simulink model "sampleModel54"  (R2021a)
settings: Solver=VariableStepAuto  StartTime=0.0  StopTime=10.0  RelTol=1e-3
libraries: simulink x28, simulink_need_slupdate x2
settings Model: Creator=user  LastModifiedBy=user

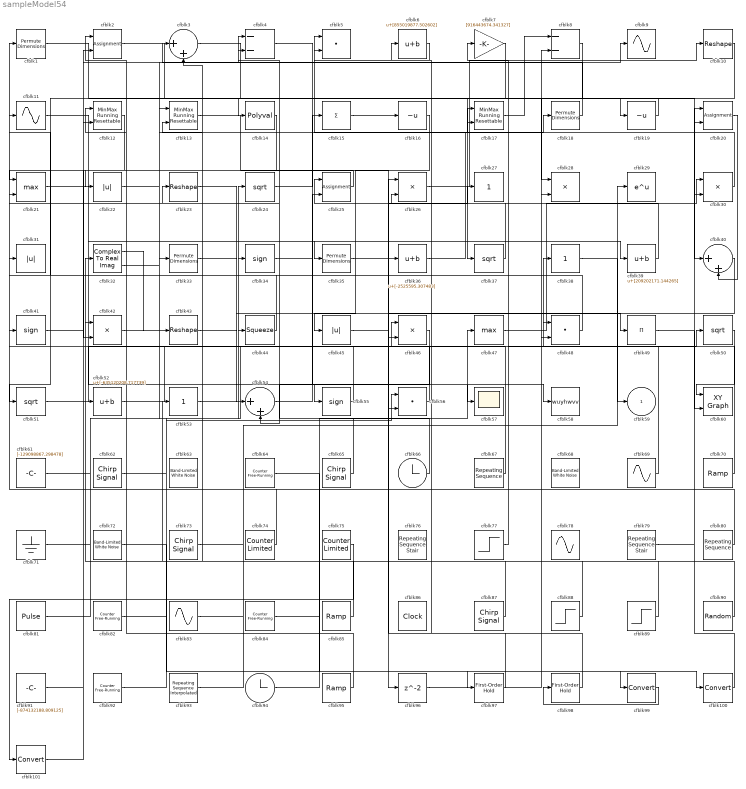
== system sampleModel54 ==
  cfblk{1,18,33,35} (4 alike) : PermuteDimensions
  cfblk10 : Reshape
  cfblk100 : DataTypeConversion
  cfblk101 : DataTypeConversion
  cfblk11 : Sin  TimeSource=Use external signal  SampleTime=0
  cfblk12 : simulink/Math Operations/MinMax Running Resettable  Function=min  vinit=0.0
  cfblk13 : simulink/Math Operations/MinMax Running Resettable  Function=min  vinit=0.0
  cfblk14 : Polyval  Coefs=[ +2.081618890e-019, -1.441693666e-014, +4.719686976e-010, -8.536869453e-006, +1.621573104e-001, -8.087801117e+001 ]
  cfblk15 : Sum  Inputs=+
  cfblk16 : UnaryMinus
  cfblk17 : simulink/Math Operations/MinMax Running Resettable  Function=min  vinit=0.0
  cfblk19 : UnaryMinus
  cfblk2 : Assignment  DiagnosticForDimensions=Warning  IndexOptions=Index vector (dialog)  Indices=1  OutputSizes=1
  cfblk20 : Assignment  DiagnosticForDimensions=Warning  IndexOptions=Index vector (dialog)  Indices=1  OutputSizes=1
  cfblk21 : MinMax  Function=max  Inputs=2
  cfblk22 : Abs
  cfblk23 : Reshape
  cfblk{24,37,50..51} (4 alike) : Sqrt  SaturateOnIntegerOverflow=on
  cfblk25 : Assignment  DiagnosticForDimensions=Warning  IndexOptions=Index vector (dialog)  Indices=1  OutputSizes=1
  cfblk26 : Product  Inputs=**
  cfblk27 : simulink/Math Operations/Slider Gain  gain=1  low=0  high=2
  cfblk28 : Product  Inputs=**
  cfblk29 : Math  SaturateOnIntegerOverflow=on
  cfblk3 : Sum  Inputs=|++
  cfblk30 : Product  Inputs=**
  cfblk31 : Abs
  cfblk32 : ComplexToRealImag
  cfblk34 : Signum
  cfblk36 : Bias  Bias=[-2525595.307483]
  cfblk38 : simulink/Math Operations/Slider Gain  gain=1  low=0  high=2
  cfblk39 : Bias  Bias=[209202171.144265]
  cfblk4 : Sum  Inputs=--
  cfblk40 : Sum  Inputs=|++
  cfblk41 : Signum
  cfblk42 : Product
  cfblk43 : Reshape
  cfblk44 : Squeeze
  cfblk45 : Abs
  cfblk46 : Product
  cfblk47 : MinMax  Function=max
  cfblk48 : DotProduct  InputSameDT=on  OutDataTypeStr=Inherit: Inherit via internal rule
  cfblk49 : Product  Inputs=*
  cfblk5 : DotProduct  InputSameDT=on  OutDataTypeStr=Inherit: Inherit via internal rule
  cfblk52 : Bias  Bias=[-635120208.717739]
  cfblk53 : simulink/Math Operations/Slider Gain  gain=1  low=0  high=2
  cfblk54 : Sum  Inputs=|++
  cfblk55 : Signum
  cfblk56 : DotProduct  InputSameDT=on  OutDataTypeStr=Inherit: Inherit via internal rule
  cfblk57 : Scope
  cfblk58 : ToWorkspace  VariableName=wuyhwvv  SaveFormat=Timeseries  SampleTime=-1
  cfblk6 : Bias  Bias=[855019877.502602]
  cfblk60 : simulink/Sinks/XY Graph  xmin=-1  xmax=1  ymin=-1  ymax=1  st=-1
  cfblk61 : Constant  Value=[-129098867.298478]  SampleTime=1
  cfblk62 : simulink/Sources/Chirp Signal  f1=[827194272.100725]  T=[195445580.820908]  f2=[-986257873.363140]
  cfblk63 : simulink/Sources/Band-Limited White Noise  Cov=[2723385097.349014]  Ts=0.1  seed=[1374667729.000000]
  cfblk64 : simulink/Sources/Counter Free-Running  NumBits=[42.000000]  tsamp=-1
  cfblk65 : simulink/Sources/Chirp Signal  f1=[-916985926.712173]  T=[-126511661.542243]  f2=[360713620.554140]
  cfblk66 : Clock
  cfblk67 : simulink/Sources/Repeating Sequence  rep_seq_t=[0 2]  rep_seq_y=[103482826.993319, -644119593.154914]
  cfblk68 : simulink/Sources/Band-Limited White Noise  Cov=[855453248.114143]  Ts=0.1  seed=[1867719781.000000]
  cfblk69 : Sin  Amplitude=[-262471217.949287]  Bias=[862179411.035081]  SampleTime=0
  cfblk7 : Gain  Gain=[916443674.341327]
  cfblk70 : simulink/Sources/Ramp  slope=[3932.769162]  start=[9.150798]  InitialOutput=[547001.441569]
  cfblk71 : Ground
  cfblk72 : simulink/Sources/Band-Limited White Noise  Cov=[4132023286.465411]  Ts=0.1  seed=[7086134090.000000]
  cfblk73 : simulink/Sources/Chirp Signal  f1=[-335725080.064148]  T=[102116674.998489]  f2=[992936377.778920]
  cfblk74 : simulink/Sources/Counter Limited  uplimit=[667.000000]  tsamp=-1
  cfblk75 : simulink/Sources/Counter Limited  uplimit=[889.000000]  tsamp=-1
  cfblk76 : simulink/Sources/Repeating Sequence Stair  OutValues=[-283484264.083720, -131969925.377744]  tsamp=-1  OutMin=[]  OutMax=[]  OutDataTypeStr=double  OutputDataTypeScalingMode=double  OutDataType=fixdt(0,8)  ConRadixGroup=Best Precision: Vector-wise  OutScaling=2^-12
  cfblk77 : Step  Time=[36.000000]  Before=[989057779.543785]  After=[-46709576.045913]  SampleTime=0
  cfblk78 : Sin  Amplitude=[-336883063.449002]  Bias=[210689002.238344]  SampleTime=0
  cfblk79 : simulink/Sources/Repeating Sequence Stair  OutValues=[546315568.995112, -228705919.390251]  tsamp=-1  OutMin=[]  OutMax=[]  OutDataTypeStr=double  OutputDataTypeScalingMode=double  OutDataType=fixdt(0,8)  ConRadixGroup=Best Precision: Vector-wise  OutScaling=2^-12
  cfblk8 : Sum  Inputs=--
  cfblk80 : simulink/Sources/Repeating Sequence  rep_seq_t=[0 2]  rep_seq_y=[-592273390.663072, -226651911.335404]
  cfblk81 : DiscretePulseGenerator  PulseType=Time based  Amplitude=[-869936793.889867]  Period=[43231919.302582]  PulseWidth=5  PhaseDelay=[7.000000]
  cfblk82 : simulink/Sources/Counter Free-Running  NumBits=[30.000000]  tsamp=-1
  cfblk83 : Sin  Amplitude=[433834177.489895]  Bias=[-397566710.558614]  SampleTime=0
  cfblk84 : simulink/Sources/Counter Free-Running  NumBits=[42.000000]  tsamp=-1
  cfblk85 : simulink/Sources/Ramp  slope=[8304.140001]  start=[35.584105]  InitialOutput=[-733753.096789]
  cfblk86 : DigitalClock
  cfblk87 : simulink/Sources/Chirp Signal  f1=[330932669.990121]  T=[-248870106.627554]  f2=[4883742.246181]
  cfblk88 : Step  Time=[20.000000]  Before=[920870307.324971]  After=[-768652709.537923]  SampleTime=0
  cfblk89 : Step  Time=[28.000000]  Before=[-65548616.125370]  After=[-682126171.802981]  SampleTime=0
  cfblk9 : Sin  TimeSource=Use external signal  SampleTime=0
  cfblk90 : UniformRandomNumber  Minimum=[-4748022415.403763]  Maximum=[3197398352.408348]  Seed=[78134240.000000]  SampleTime=0.1
  cfblk91 : Constant  Value=[-874132188.809125]  SampleTime=1
  cfblk92 : simulink/Sources/Counter Free-Running  NumBits=[38.000000]  tsamp=-1
  cfblk93 : simulink/Sources/Repeating Sequence Interpolated  OutValues=[-837789551.832010, 692628790.459985, 723871985.487427, 517447538.050501, 875468418.107600]  TimeValues=[0 0.1 0.5 0.6 1].'  LookUpMeth=Use Input Below  tsamp=0.01  OutMin=[]  OutMax=[]  OutDataTypeStr=double  OutputDataTypeScalingMode=double  OutDataType=fixdt(0,8)  OutScaling=2^-10
  cfblk94 : Clock
  cfblk95 : simulink/Sources/Ramp  slope=[9920.536367]  start=[37.074568]  InitialOutput=[-885041.909920]
  cfblk96 : Delay  SampleTime=1
  cfblk97 : simulink_need_slupdate/First-Order Hold  DisableCoverage=on  Ts=1
      settings: SourceProductBaseCode=SL
  cfblk98 : simulink_need_slupdate/First-Order Hold  DisableCoverage=on  Ts=1
      settings: SourceProductBaseCode=SL
  cfblk99 : DataTypeConversion
  cfblk59 : Outport
  wires:
  cfblk80/1 -> cfblk1/1
  cfblk25/1 -> cfblk21/1
  cfblk17/1 -> cfblk8/1
  cfblk81/1 -> cfblk24/1
  cfblk94/1 -> cfblk47/1
  cfblk32/1 -> cfblk43/1
  cfblk71/1 -> cfblk33/1
  cfblk11/1 -> cfblk57/1
  cfblk32/2 -> cfblk13/1
  cfblk2/1 -> cfblk40/1
  cfblk47/1 -> cfblk30/1
  cfblk88/1 -> cfblk23/1
  cfblk50/1 -> cfblk60/1
  cfblk21/1 -> cfblk35/1
  cfblk23/1 -> cfblk49/1
  cfblk61/1 -> cfblk34/1
  cfblk74/1 -> cfblk32/1
  cfblk92/1 -> cfblk44/1
  cfblk51/1 -> cfblk46/1
  cfblk53/1 -> cfblk36/1
  cfblk38/1 -> cfblk59/1
  cfblk20/1 -> cfblk40/2
  cfblk13/1 -> cfblk46/2
  cfblk30/1 -> cfblk5/1
  cfblk15/1 -> cfblk16/1
  cfblk95/1 -> cfblk12/1
  cfblk44/1 -> cfblk31/1
  cfblk91/1 -> cfblk12/2
  cfblk66/1 -> cfblk42/1
  cfblk42/1 -> cfblk9/1
  cfblk8/1 -> cfblk51/1
  cfblk82/1 -> cfblk50/1
  cfblk6/1 -> cfblk5/2
  cfblk41/1 -> cfblk4/1
  cfblk33/1 -> cfblk54/1
  cfblk12/1 -> cfblk22/1
  cfblk52/1 -> cfblk38/1
  cfblk14/1 -> cfblk42/2
  cfblk43/1 -> cfblk55/1
  cfblk37/1 -> cfblk6/1
  cfblk89/1 -> cfblk53/1
  cfblk87/1 -> cfblk2/1
  cfblk62/1 -> cfblk56/1
  cfblk39/1 -> cfblk25/1
  cfblk10/1 -> cfblk19/1
  cfblk46/1 -> cfblk54/2
  cfblk70/1 -> cfblk48/1
  cfblk55/1 -> cfblk13/2
  cfblk85/1 -> cfblk52/1
  cfblk4/1 -> cfblk58/1
  cfblk40/1 -> cfblk56/2
  cfblk18/1 -> cfblk3/1
  cfblk19/1 -> cfblk14/1
  cfblk79/1 -> cfblk30/2
  cfblk67/1 -> cfblk41/1
  cfblk7/1 -> cfblk37/1
  cfblk3/1 -> cfblk20/2
  cfblk34/1 -> cfblk39/1
  cfblk73/1 -> cfblk29/1
  cfblk26/1 -> cfblk10/1
  cfblk48/1 -> cfblk11/1
  cfblk36/1 -> cfblk18/1
  cfblk1/1 -> cfblk28/1
  cfblk24/1 -> cfblk15/1
  cfblk83/1 -> cfblk28/2
  cfblk65/1 -> cfblk21/2
  cfblk45/1 -> cfblk27/1
  cfblk69/1 -> cfblk7/1
  cfblk90/1 -> cfblk3/2
  cfblk16/1 -> cfblk45/1
  cfblk49/1 -> cfblk60/2
  cfblk93/1 -> cfblk48/2
  cfblk56/1 -> cfblk4/2
  cfblk22/1 -> cfblk17/1
  cfblk77/1 -> cfblk17/2
  cfblk54/1 -> cfblk25/2
  cfblk35/1 -> cfblk96/1
  cfblk96/1 -> cfblk8/2
  cfblk72/1 -> cfblk97/1
  cfblk97/1 -> cfblk26/1
  cfblk98/1 -> cfblk26/2
  cfblk64/1 -> cfblk99/1
  cfblk99/1 -> cfblk98/1
  cfblk84/1 -> cfblk100/1
  cfblk100/1 -> cfblk20/1
  cfblk75/1 -> cfblk101/1
  cfblk101/1 -> cfblk2/2
